simulink model "CTRL_BASECTRL_SKY_test"  (R2024b)
settings: Solver=VariableStepAuto  StartTime=0.0  StopTime=10.0  RelTol=1e-3
libraries: CTRL_BASECTRL_SKY x1
settings Model: Creator=blatak  LastModifiedBy=blatak

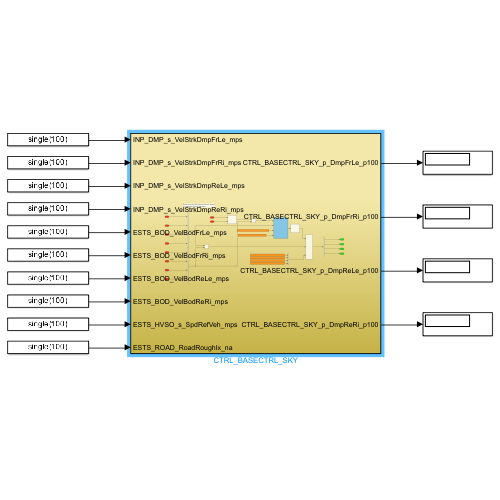
[thumbnail: Simulink's stored preview of the top-level diagram]
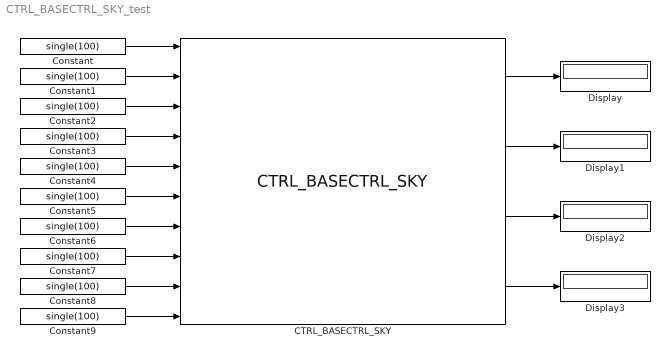
== system CTRL_BASECTRL_SKY_test ==
  CTRL_BASECTRL_SKY : CTRL_BASECTRL_SKY/CTRL_BASECTRL_SKY  SystemSampleTime=-1  VariantActivationTime=update diagram  AllowFlexibleInterface=on  Latency=0  AutoFrameSizeCalculation=off
  Constant{,1..9} (10 alike) : Constant  Value=single(100)
  Display{,1..3} (4 alike) : Display
  wires:
  Constant/1 -> CTRL_BASECTRL_SKY/1
  Constant1/1 -> CTRL_BASECTRL_SKY/2
  Constant2/1 -> CTRL_BASECTRL_SKY/3
  Constant3/1 -> CTRL_BASECTRL_SKY/4
  Constant4/1 -> CTRL_BASECTRL_SKY/5
  Constant5/1 -> CTRL_BASECTRL_SKY/6
  Constant6/1 -> CTRL_BASECTRL_SKY/7
  Constant7/1 -> CTRL_BASECTRL_SKY/8
  Constant8/1 -> CTRL_BASECTRL_SKY/9
  Constant9/1 -> CTRL_BASECTRL_SKY/10
  CTRL_BASECTRL_SKY/1 -> Display/1
  CTRL_BASECTRL_SKY/2 -> Display1/1
  CTRL_BASECTRL_SKY/3 -> Display2/1
  CTRL_BASECTRL_SKY/4 -> Display3/1
